simulink model "MicroMouseTemplate"  (R2024a)
settings: Solver=FixedStepAuto  StartTime=0.0  StopTime=10.0  RelTol=1e-3  EnableMultiTasking=on
undefined symbols (not defined in the file): samplingTime
settings Model: STM32="{\"DigitalPortWrite\":[{\"ID\":\"MicroMouseTemplate:84:3\"},{\"ID\":\"MicroMouseTemplate:84:4\"},{\"ID\":\"MicroMouseTemplate:84:5\"},{\"ID\":\"MicroMouseTemplate:84:6\"},{\"ID\":\"MicroMouseTemplate:84:7\"},{\"ID\":\"MicroMouseTemplate:84:8\"},{\"ID\":\"MicroMouseTemplate:84:9\"},{\"ID\":\"MicroMouseTemplate:84:10\"},{\"ID\":\"MicroMouseTemplate:160:19\"},{\"ID\":\"MicroMouseTemplate:2479:4\"},{\"ID\":\"MicroMouseTemplate:2479:6\"},{\"ID\":\"MicroMouseTemplate:2479:7\"},{\"ID\":\"MicroMouseTemplate:2479:8\"}],\"PWMOutput\":[{\"ID\":\"MicroMouseTemplate:160:24\"},{\"ID\":\"MicroMouseTemplate:160:25\"}],\"AnalogInput\":{\"ID\":\"MicroMouseTemplate:2357:1\"},\"DigitalPortRead\":[{\"ID\":\"MicroMouseTemplate:2483:3\"},{\"ID\":\"MicroMouseTemplate:2483:4\"}]}"  ExtModeTrigDuration=10  Creator=JesseJabezArendse  LastModifiedBy=griff
settings SolverCC: AllowMultiTaskInputOutput=on  AutoInsertRateTranBlk=on  InsertRTBMode=Never (minimum delay)
settings OptimizationCC: EnhancedBackFolding=on  PassReuseOutputArgsAs=Individual arguments  StateBitsets=on  DataBitsets=on  ZeroExternalMemoryAtStartup=off  ZeroInternalMemoryAtStartup=off  NoFixptDivByZeroProtection=on  MaxStackSize=64  OptimizeBlockOrder=speed  DifferentSizesBufferReuse=on  EfficientTunableParamExpr=on
settings DebuggingCC: MultiTaskCondExecSysMsg=none  ParameterOverflowMsg=none  ParameterPrecisionLossMsg=none  ParameterTunabilityLossMsg=error
settings HardwareCC: ProdBitPerPointer=32  ProdBitPerSizeT=32  ProdBitPerPtrDiffT=32  ProdLargestAtomicInteger=Long  ProdLargestAtomicFloat=Double  ProdWordSize=32  ProdLongLongMode=on  ProdHWDeviceType=ARM Compatible->ARM Cortex  TargetBitPerPointer=64  TargetBitPerSizeT=64  TargetBitPerPtrDiffT=64  TargetLongLongMode=on  TargetIntDivRoundTo=Zero  TargetEndianess=LittleEndian  TargetWordSize=64  TargetHWDeviceType=MATLAB Host
settings ModelReferenceCC: EnableParallelModelReferenceBuilds=on  ParallelModelReferenceMATLABWorkerInit=Copy Base Workspace  SupportModelReferenceSimTargetCustomCode=on
settings SFSimCC: MATLABDynamicMemAlloc=off  SimHardwareAcceleration=native
settings RTWCC: Description=Embedded Coder  SystemTargetFile=ert.tlc  HardwareBoard=STM32L4xx Based  TLCOptions=-p0 -aInlineSetEventsForThisBaseRateFcn=TLC_FALSE -aSuppressMultiTaskScheduler=TLC_FALSE -aRateBasedStepFcn=1  TemplateMakefile=ert_default_tmf  Toolchain=GNU Tools for ARM Embedded Processors  BuildConfiguration=Faster Runs  CodeExecutionProfiling=on  CodeProfilingInstrumentation=coarse  GPUComputeCapability=3.5
settings RTWCC: CustomHeaderCode=|
  | #include "MicroMouseProgramming\Core\Inc\IMU.h"
  | #include "MicroMouseProgramming\Core\Inc\CustomWhile.h"
  | #include "MicroMouseProgramming\Core\Inc\Motors.h"
settings RTWCC: CustomInclude=|
  | MicroMouseProgramming\Core\Inc\
  | MicroMouseProgramming\Core\Src\
settings RTWCC: CustomSource=|
  | MicroMouseProgramming\Core\Src\IMU.c
  | MicroMouseProgramming\Core\Src\CustomWhile.c
  | MicroMouseProgramming\Core\Src\Motors.c
settings CodeAppCC: GenerateComments=off  IgnoreCustomStorageClasses=off  OperatorAnnotations=on  SimulinkDataObjDesc=on  SFDataObjDesc=on  SimulinkBlockComments=off
settings ERTTargetCC: CodeReplacementLibrary=ARM Cortex-M  SupportNonFinite=off  SupportComplex=off  SupportVariableSizeSignals=on  ExtModeTransport=3  ExtModeStaticAlloc=on  ExtModeStaticAllocSize=2048  ExtModeMexFile=ext_xcp  ExtModeIntrfLevel=Level2 - Open

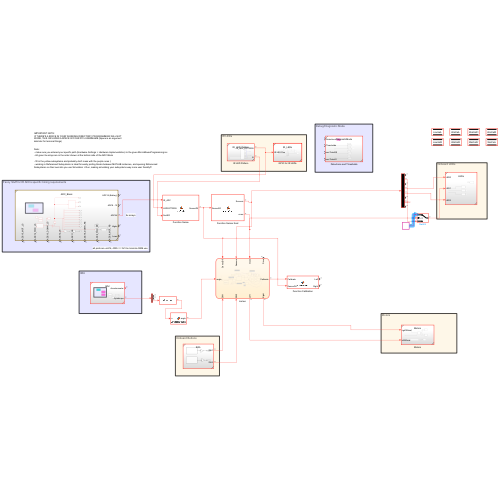
[thumbnail: Simulink's stored preview of the top-level diagram]
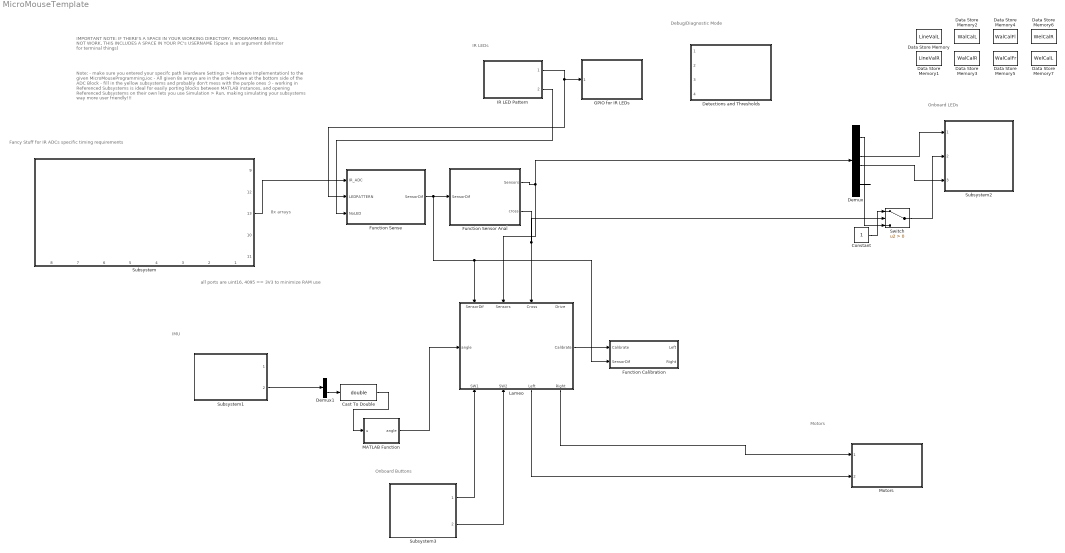
== system MicroMouseTemplate ==
  note: IMPORTANT NOTE:
      | IF THERE'S A SPACE IN YOUR WORKING DIRECTORY, PROGRAMMING WILL NOT WORK, THIS INCLUDES A SPACE IN YOUR PC's USERNAME (Space is an argument delimiter for terminal things)
  note: Note:
      | - make sure you entered your specifc path (Hardware Settings > Hardware Implementation) to the given MicroMouseProgramming.ioc
      | - All given 8x arrays are in the order shown at the bottom side of the ADC Block
      |
      | - fill in the yellow subsystems and probably don't mess with the purple ones :)
      | - working in Referenced Subsystems is ideal for easily porting blocks between MATLAB instances, and opening Referenced Subsystems on their own lets you use Simulation > Run, making simulating your subsystems way more user friendly!!!
  note: 8x arrays
  note: all ports are uint16, 4095 == 3V3 to minimize RAM use
  note: IMU
  note: Fancy Stuff for IR ADCs specific timing requirements
  note: IR LEDs
  note: Motors
  note: Onboard Buttons
  note: Onboard LEDs
  note: Debug/Diagnostic Mode
  Cast To Double : DataTypeConversion  OutDataTypeStr=double  SaturateOnIntegerOverflow=off  RndMeth=Floor
  Constant : Constant
  Data Store Memory : DataStoreMemory  DataStoreName=LineValL  WriteAfterWriteMsg=warning  ShowAdditionalParam=off  OutDataTypeStr=double
  Data Store Memory1 : DataStoreMemory  DataStoreName=LineValR  WriteAfterWriteMsg=warning  ShowAdditionalParam=off  OutDataTypeStr=double
  Data Store Memory2 : DataStoreMemory  DataStoreName=WalCalL  WriteAfterWriteMsg=warning  ShowAdditionalParam=off  OutDataTypeStr=double
  Data Store Memory3 : DataStoreMemory  DataStoreName=WalCalR  WriteAfterWriteMsg=warning  ShowAdditionalParam=off  OutDataTypeStr=double
  Data Store Memory4 : DataStoreMemory  DataStoreName=WalCalFl  WriteAfterWriteMsg=warning  ShowAdditionalParam=off  OutDataTypeStr=double
  Data Store Memory5 : DataStoreMemory  DataStoreName=WalCalFr  WriteAfterWriteMsg=warning  ShowAdditionalParam=off  OutDataTypeStr=double
  Data Store Memory6 : DataStoreMemory  DataStoreName=WelCalR  WriteAfterWriteMsg=warning  ShowAdditionalParam=off  OutDataTypeStr=double
  Data Store Memory7 : DataStoreMemory  DataStoreName=WelCalL  WriteAfterWriteMsg=warning  ShowAdditionalParam=off  OutDataTypeStr=double
  Demux : Demux  Outputs=8
  Demux1 : Demux  Outputs=3
  Detections and Thresholds : Subsystem  ReferencedSubsystem=DiagnosticMode
  Function Calibration : MATLAB Function  TreatAsAtomicUnit=on
  Function Sense : MATLAB Function  TreatAsAtomicUnit=on
  Function Sensor Anal : MATLAB Function  TreatAsAtomicUnit=on
  GPIO for IR LEDs : Subsystem  TreatAsAtomicUnit=on  SystemSampleTime=samplingTime  ReferencedSubsystem=IR_LEDs
  IR LED Pattern : Subsystem  ReferencedSubsystem=IR_LED_Pattern
  Lameo : Stateflow chart  TreatAsAtomicUnit=on
      settings: PortSchema="{\"entries\":[{\"content\":{\"sides\":[{\"content\":{\"connectorIds\":[\"In2\"]},\"type\":\"ConnectorPlacement.EquallySpacedRectSide\",\"uuid\":\"f52daa4f-6374-42e5-9ef1-0ccc99d09b58\"},{\"content\":{\"connectorIds\":[\"Out1\"],\"side\":\"RIGHT\"},\"type\":\"ConnectorPlacement.EquallySpacedRectSide\",\"uuid\":\"94b478cc-4dde-45c7-a588-77cf2b43cdb7\"},{\"content\":{\"connectorIds\":[\"In1\",\"In3\",\"In4\",\"Out2\"],\"side\":\"TOP\"},\"type\":\"ConnectorPlacement.EquallySpacedRectSide\",\"uuid\":\"afff2079-ea5c-423e-9722-09c3bbce433b\"},{\"content\":{\"connectorIds\":[\"In6\",\"In5\",\"Out3\",\"Out4\"],\"side\":\"BOTTOM\"},\"type\":\"ConnectorPlacement.EquallySpacedRectSide\",\"uuid\":\"94e93a1d-795d-41a3-b2d8-d520b2bf47ef\"}]},\"type\":\"ConnectorPlacement.EquallySpacedConnector\",\"uuid\":\"d4d35636-54af-48ac-af70-d56caef5e090\"}],\"packageUris\":[\"http://schema.mathworks.com/mf0/Connector/R2020b\"],\"version\":\"1.0\"}"
  MATLAB Function : MATLAB Function  TreatAsAtomicUnit=on
  Motors : Subsystem  ReferencedSubsystem=Motors
  Subsystem : Subsystem  ReferencedSubsystem=ADC_Block
      settings: PortSchema="{\"entries\":[{\"content\":{\"sides\":[{\"content\":{},\"type\":\"ConnectorPlacement.EquallySpacedRectSide\",\"uuid\":\"be6b81d5-7a49-4e34-b35f-0c07892094fc\"},{\"content\":{\"connectorIds\":[\"Out1\",\"Out2\",\"Out3\",\"Out4\",\"Out5\",\"Out6\",\"Out7\",\"Out8\"],\"side\":\"RIGHT\"},\"type\":\"ConnectorPlacement.EquallySpacedRectSide\",\"uuid\":\"5e22590a-b7c0-4c63-8de4-8d81fd6c3849\"},{\"content\":{\"connectorIds\":[\"Out9\",\"Out12\",\"Out13\",\"Out10\",\"Out11\"],\"side\":\"TOP\"},\"type\":\"ConnectorPlacement.EquallySpacedRectSide\",\"uuid\":\"da97636e-cea0-4a10-8fe5-d807f9ee999f\"},{\"content\":{\"side\":\"BOTTOM\"},\"type\":\"ConnectorPlacement.EquallySpacedRectSide\",\"uuid\":\"a593d780-81a8-4730-a8bc-2bbf356cafe4\"}]},\"type\":\"ConnectorPlacement.EquallySpacedConnector\",\"uuid\":\"0bcac921-e51a-4437-9183-315712d0a8c2\"}],\"packageUris\":[\"http://schema.mathworks.com/mf0/Connector/R2020b\"],\"version\":\"1.0\"}"
  Subsystem1 : Subsystem  ReferencedSubsystem=IMU
  Subsystem2 : Subsystem  ReferencedSubsystem=LEDs
  Subsystem3 : Subsystem  ReferencedSubsystem=SWs
  Switch : Switch  Criteria=u2 > Threshold  SaturateOnIntegerOverflow=off  InputSameDT=off
  wires:
  Subsystem3/1 -> Lameo/6(SW1)
  Subsystem3/2 -> Lameo/5(SW2)
  IR LED Pattern/1 -> Function Sense/2(LEDPATTERN), GPIO for IR LEDs/1
  Subsystem/13 -> Function Sense/1(IR_ADC)
  IR LED Pattern/2 -> Function Sense/3(NoLED)
  Function Sense/1(SensorDif) -> Lameo/1(SensorDif), Function Calibration/2(SensorDif), Function Sensor Anal/1(SensorDif)
  Lameo/1(Calibrate) -> Function Calibration/1(Calibrate)
  Lameo/3(Left) -> Motors/2
  Lameo/4(Right) -> Motors/1
  Function Sensor Anal/1(Sensors) -> Lameo/3(Sensors), Demux/1
  Function Sensor Anal/2(cross) -> Switch/2, Lameo/4(Cross)
  Subsystem1/2 -> Demux1/1
  Demux1/3 -> Cast To Double/1
  Cast To Double/1 -> MATLAB Function/1(u)
  MATLAB Function/1(angle) -> Lameo/2(angle)
  Demux/2 -> Switch/3
  Demux/7 -> ?
  Demux/4 -> Subsystem2/1
  Demux/5 -> Subsystem2/3
  Constant/1 -> Switch/1
  Switch/1 -> Subsystem2/2

== matlab function MicroMouseTemplate/Function Calibration ==
  data: Calibrate input; Left output; Right output; LineValR data_store_memory; SensorDif input; LineValL data_store_memory; WalCalR data_store_memory; WalCalL data_store_memory; WalCalFr data_store_memory; WalCalFl data_store_memory; WelCalL data_store_memory; WelCalR data_store_memory
function [Left,Right]  = Calbiration(Calibrate, SensorDif)


persistent mindl
if isempty(mindl)
    mindl = 3;
end
persistent maxdl
if isempty(maxdl)
    maxdl = 0;
end
persistent mindr
if isempty(mindr)
    mindr = 3;
end
persistent maxdr
if isempty(maxdr)
    maxdr = 0;
end



persistent minwl
if isempty(minwl)
    minwl = 3;
end
persistent maxwl
if isempty(maxwl)
    maxwl = 0;
end

persistent minwfr
if isempty(minwfr)
    minwfr = 3;
end
persistent maxwfr
if isempty(maxwfr)
    maxwfr = 0;
end
persistent minwfl
if isempty(minwfl)
    minwfl = 3;
end
persistent maxwfl
if isempty(maxwfl)
    maxwfl = 0;
end

persistent minwr
if isempty(minwr)
    minwr = 3;
end
persistent maxwr
if isempty(maxwr)
    maxwr = 0;
end

persistent minwer
if isempty(minwer)
    minwer = 3;
end
persistent maxwer
if isempty(maxwer)
    maxwer = 0;
end
persistent minwel
if isempty(minwel)
    minwel = 3;
end
persistent maxwel
if isempty(maxwel)
    maxwel = 0;
end






Left=0;
Right=0;
if Calibrate==1
    Right=75;
    Left=-75;
    if SensorDif(3)>(maxdl)
        maxdl=maxdl*0.8+0.2*SensorDif(3);
    end
    if SensorDif(3)<(mindl)
        mindl=mindl*0.8+0.2*SensorDif(3);
    end
    if SensorDif(6)>(maxdr)
        maxdr=maxdr*0.8+0.2*SensorDif(6);
    end
    if SensorDif(6)<(mindr)
        mindr=mindr*0.8+0.2*SensorDif(6);
    end

    if SensorDif(4)>(maxwr)
        maxwr=maxwr*0.5+0.5*SensorDif(4);
    end
    if SensorDif(4)<(minwr)
        minwr=minwr*0.5+0.5*SensorDif(4);
    end
    if SensorDif(5)>(maxwl)
        maxwl=maxwl*0.5+0.5*SensorDif(5);
    end
    if SensorDif(5)<(minwl)
        minwl=minwl*0.5+0.5*SensorDif(5);
    end

    if (SensorDif(2))>(maxwfr)
        maxwfr=maxwfr*0.5+0.5*(SensorDif(2));
    end
    if (SensorDif(2))<(minwfr)
        minwfr=minwfr*0.5+0.5*(SensorDif(2));
    end
    if (SensorDif(7))>(maxwfl)
        maxwfl=maxwfl*0.5+0.5*(SensorDif(7));
    end
    if (SensorDif(7))<(minwfl)
        minwfl=minwfl*0.5+0.5*(SensorDif(7));
    end


     if SensorDif(1)>(maxwer)
        maxwer=maxwer*0.8+0.2*SensorDif(1);
    end
    if SensorDif(1)<(minwer)
        minwer=minwer*0.8+0.2*SensorDif(1);
    end
    if SensorDif(8)>(maxwel)
        maxwel=maxwel*0.8+0.2*SensorDif(8);
    end
    if SensorDif(8)<(minwel)
        minwel=minwel*0.8+0.2*SensorDif(8);
    end


end



global LineValR
LineValR=(maxdr-mindr)*0.7+mindr;%(mindr+maxdr)/2*1.1;
global LineValL
LineValL=(maxdl-mindl)*0.7+mindl;%(mindl+maxdl)/2*1.1;

global WalCalL
WalCalL=(maxwl-minwl)*0.4+minwl;%(minwl+maxwl)/2;
%WalCalL=((maxwl)*0.85);
global WalCalR
WalCalR=(maxwr-minwr)*0.4+minwr;%(minwr+maxwr)/2;
%WalCalR=((maxwr)*0.85);
global WalCalFl
%WalCalFl=(minwfl+maxwfl)/2;
WalCalFl=(maxwfl-minwfl)*0.3+minwfl;%((maxwfl)*0.6);
global WalCalFr
%WalCalFr=(minwfr+maxwfr)/2;
WalCalFr=(maxwfr-minwfr)*0.3+minwfr;%((maxwfr)*0.6);

global WelCalL
WelCalL=(maxwel-minwel)*0.8+minwel;
global WelCalR
WelCalR=(maxwer-minwer)*0.8+minwer;

end

== stateflow chart MicroMouseTemplate/Lameo ==
  state Crossing
    entry:
    Turn =thingy;
    pos(1)=pos(1)+direction(2)-direction(4);
    pos(2)=pos(2)+direction(1)-direction(3);
  state Calibration
    during:
    Calibrate =1 ;
    Right=50;
    Left=-50;
  state Delay
  state Center
    during:
    [Left,Right]=CenterLine(1,Sensors)
    Calibrate =0;
  state Back
    during:
    Left=-50;
    Right=-50;
  state Back2
    during:
    Left=-50;
    Right=-50;
  state Back1
    during:
    Left=-50;
    Right=-50;
  state OK
    entry:
    temp=start
    start=dest
    dest=temp
    Left=0;
    Right=0;
  state TurnRight
    entry:
    Left=100;
    Right=-50;
    DesA=angle-90;
    exit:
    Left=0;
    Right=0;
    res=1;
  state TurnLeft
    entry:
    Left=-50;
    Right=100;
    DesA=angle+90;
    exit:
    Left=0;
    Right=0;
    res=1;
  state Flip
    entry:
    Left=-50;
    Right=50;
    DesA=angle+180;
    exit:
    Left=0;
    Right=0;
    res=1;
  state Idle
    entry:
    %Varibales needed for path finding
    Left=0;
    Right=0;
    pathend=0;
    %end
    during:
    Calibrate =0 ;
    Drive=0;
  state Drive
    entry:
    Drive=1;
    [Left,Right]=FollowLine(Drive,Sensors,res,SensorDif)
    during:
    [Left,Right]=FollowLine(Drive,Sensors,0,SensorDif)
  state Init1
    entry:
    Init;
    start=int16([1;1]);
    pos=start;
    dest=int16([2;1]);
    direction= int16([1;0;0;0]);
    desA=0;
  state Wait
  state TurnWrong
    entry:
    Left=-50;
    Right=50;
    exit:
    Left=0;
    Right=0;
  state TurnWrong1
    entry:
    Left=50;
    Right=-50;
    exit:
    Left=0;
    Right=0;
  state TurnWrong2
    entry:
    Left=50;
    Right=-50;
    exit:
    Left=0;
    Right=0;
  state Hehehehe
    state T
      during:
      Left=100;
      Right=-100;
    state TT
      during:
      Left=-100;
      Right=100;
    (default) -> T
    TT -> T : after(0.02,sec)
    T -> TT : after(0.02,sec)
  state Mistake
    entry:
    delConnection(pos(1),pos(2),pos(1)+direction(2)-direction(4),pos(2)+direction(1)-direction(3))
    direction= circshift(direction,2);
    pos(1)=pos(1)+direction(2)-direction(4);
    pos(2)=pos(2)+direction(1)-direction(3)
  state TEst
    entry:
    desA=desA+90;
    during:
    [Left,Right]=CenterAngle(angle,desA)
  OK -> Delay : after(2,sec)
  Delay -> Crossing : after(1,sec)
  Crossing -> Back [order 3] : [Turn==2]
  Calibration -> Center : [after(4,sec)]
  Crossing -> Back1 [order 1] : [Turn==-1]
  Idle -> Delay [order 2] : [SW1]
  Crossing -> Back2 [order 2] : [Turn==1]
  Idle -> Calibration [order 1] : [SW2&&after(2,sec)]
  Drive -> Crossing [order 2] : [Cross==1&&(after(0.4,sec))]
  (default) -> Wait
  Back -> Flip : after(0.1,sec)
  Back2 -> TurnRight : after(0.1,sec)
  Back1 -> TurnLeft : after(0.1,sec)
  Center -> Idle : after(1,sec)
  Crossing -> Drive [order 4] : [Turn==0]{res=0;}
  Drive -> OK [order 1] : [Cross==1&&(after(0.4,sec))&&(pos(1)==dest(1)&&pos(2)==dest(2))]
  Mistake -> Flip
  TurnRight -> TurnWrong : [(DesA-angle>-20)&&Sensors(6)==0]
  TurnLeft -> TurnWrong1 : [(DesA-angle<20)&&Sensors(3)==0]
  Flip -> TurnWrong2 : [(DesA-angle<10)&&Sensors(6)==0]
  Wait -> Init1 : after(1,sec)
  TurnWrong -> Drive : after(0.05,sec)
  TurnWrong1 -> Drive : after(0.05,sec)
  Hehehehe -> Init1 : after(1,sec)
  TurnWrong2 -> Drive : after(0.1,sec)
  Init1 -> Idle
  Drive -> Mistake [commented out] : [Sensors(2)==1&&before(0.3,sec)]
  TEst -> TEst : after(1,sec)
  data: Drive function_input; Sensors function_input; Left function_output; Right function_output; Drive function_input; Sensors function_input; Left function_output; Right function_output; first function_input; SensorDif function_input; x1 function_input; y1 function_input; x2 function_input; y2 function_input; Angle function_input; Setpoint function_input; Left function_output; Right function_output; Turn function_output; SensorDif input; angle input; Sensors input; Cross input; SW2 input; SW1 input; Calibrate output; Drive output; Left output; Right output; Turn local; numH local int16 size=1; numV local int16 size=1; pos local int16 size=2; dest local int16 size=2; direction local int16 size=4; connection local int16 size=168 4; connectionend local int16 size=1; dist local int16 size=[7 7]; path local int16 size=200 2; pre local int16 size=7 7 2; q local int16 size=200 2; qend local int16 size=1; pathend local int16 size=1; start local; temp local; desA local; DesA local; LineValR data_store_memory; LineValL data_store_memory; res local
  function [Left,Right] = CenterLine(Drive, Sensors):
    | function [Left,Right] = CenterLine(Drive, Sensors)
    | P = 10;
    | I =0.5;
    | D=50;
    | 
    | 
    | persistent preError
    | if isempty(preError)
    |     preError=0;
    | end
    | persistent sumError
    | if isempty(sumError)
    |     sumError=0;
    | end
    | persistent error
    | if isempty(error)
    |     error=0;
    | end
    | persistent Dave
    | if isempty(Dave)
    |     Dave=0;
    | end
    | 
    | 
    | 
    | Left=0;
    | Right=0;
    | 
    | if Drive ==1
    | Left=0;
    | Right=0;
    | 
    | 
    | if (Sensors(3)==1&&Sensors(6)==0)
    |     error=-1;   
    | end
    | if (Sensors(3)==0&&Sensors(6)==1)
    |     error=1;   
    | end
    | if (Sensors(3)==0&&Sensors(6)==0)
    |     error=0;   
    | end
    | if (error==1&&Sensors(3)==1&&Sensors(6)==1)
    |     error=2;  
    | end
    | if (error==-1&&Sensors(3)==1&&Sensors(6)==1)
    |     error=-2; 
    | end
    | 
    | sumError=sumError+error;
    | sumError= sumError-0.005*sumError;
    | 
    | 
    | Dave=(error-preError)+0.8*Dave;
    | 
    | PID= P*error+I*sumError+D*(Dave);
    | preError=error;
    | 
    | 
    | Left=0-PID;
    | Right=0+PID;
    | Left = min(max(Left,-100),100);
    | Right = min(max(Right,-100),100);
    | 
    | if (error==0&&Sensors(3)==1&&Sensors(6)==1)
    |     Left=-50;
    |     Right=-50;
    | end
    | 
    | 
    | 
    | 
    | 
    | if Sensors(2)==1
    |    % Left=0;
    |    % Right=0;
    | end
    | 
    | 
    | 
    | 
    | 
    | 
    | 
    | 
    | 
    | 
    | 
    | 
    | 
    | 
    | end
    | 
    | end
  function [Left,Right] = FollowLine(Drive, Sensors,first,SensorDif):
    | function [Left,Right] = FollowLine(Drive, Sensors,first,SensorDif)
    | P = 15;
    | I =0.5;
    | D=125;
    | global LineValL
    | global LineValR
    | 
    | 
    | 
    | persistent preError
    | if isempty(preError)
    |     preError=0;
    | end
    | persistent preSide
    | if isempty(preSide)
    |     preSide=0;
    | end
    | persistent sumError
    | if isempty(sumError)
    |     sumError=0;
    | end
    | persistent error
    | if isempty(error)
    |     error=0;
    | end
    | persistent Dave
    | if isempty(Dave)
    |     Dave=0;
    | end
    | 
    | if (first==1)
    |     Dave=0;
    |     error=0;
    |     preError=0;
    |     sumError=0;
    | end
    | 
    | Left=0;
    | Right=0;
    | 
    | if Drive ==1
    | Left=100;
    | Right=100;
    | 
    | 
    | if (Sensors(3)==1&&Sensors(6)==0)
    |     error=-1;  
    |     preSide = error;
    | end
    | if (Sensors(3)==0&&Sensors(6)==1)
    |     error=1;  
    |     preSide = error;
    | end
    | if (Sensors(3)==0&&Sensors(6)==0)
    |     error=0; 
    |    
    | end
    | if (error==1&&Sensors(3)==1&&Sensors(6)==1)
    |     error=2;  
    |     preSide = error;
    | end
    | if (error==-1&&Sensors(3)==1&&Sensors(6)==1)
    |     error=-2; 
    |     preSide = error;
    | end
    | 
    | if (error==0&&Sensors(3)==1&&Sensors(6)==1)
    |     error=-preSide;
    | end
    | 
    | 
    | sumError=sumError+error;
    | sumError= sumError-0.005*sumError;
    | 
    | 
    | Dave=(error-preError)+0.8*Dave;
    | 
    | PID= P*error+I*sumError+D*(Dave);
    | preError=error;
    | 
    | 
    | Left=100-PID;
    | Right=100+PID;
    | Left = min(max(Left,-100),100);
    | Right = min(max(Right,-100),100);
    | 
    | 
    | 
    | 
    | 
    | 
    | if Sensors(2)==1
    |    % Left=0;
    |    % Right=0;
    | end
    | 
    | 
    | 
    | 
    | 
    | 
    | 
    | 
    | 
    | 
    | 
    | 
    | 
    | 
    | end
    | 
    | end
  function Init:
    | function Init
    | global pos
    |  pos=int16([1;2]);
    |  global dest
    | dest=int16([2;1]);
    | global direction
    | direction= int16([1;0;0;0]);
    | global numH
    | numH = int16(7);
    | global numV
    | numV = int16(7);
    | global connection
    | connection = zeros(168,4,'int16');
    | global connectionend
    | connectionend=int16(0);
    | 
    | 
    | 
    | 
    | 
    | for x = 1:numH
    |        for y = 1:numV
    |             if x>1
    |             connection(connectionend+1, :) = [x, y, x-1, y];
    |             connectionend=connectionend+1;
    |             end
    |             if y>1
    |              connection(connectionend+1, :) = [x, y, x, y-1];
    |              connectionend=connectionend+1;
    |             end
    |             if x<numH
    |              connection(connectionend+1, :) = [x, y, x+1, y];
    |              connectionend=connectionend+1;
    |             end
    |             if y<numV
    |              connection(connectionend+1, :) = [x, y, x, y+1];
    |              connectionend=connectionend+1;
    |             end
    | 
    | 
    |        end
    | end
    | 
    | end
  function delConnection(x1,y1,x2,y2):
    | function delConnection(x1,y1,x2,y2)
    | global connection;
    |     for i = 1:size(connection,1)
    |         if connection(i,1) == x1 & connection(i,2) == y1 & connection(i,3) == x2 & connection(i,4) == y2
    |             connection(i,:) = [0,0,0,0];
    |         end
    |         if connection(i,1) == x2 & connection(i,2) == y2 & connection(i,3) == x1 & connection(i,4) == y1
    |             connection(i,:) = [0,0,0,0];
    |         end
    |         
    |     end
    | 
    | end
  function route:
    | function route
    |     global connection;
    |     global dist;
    |     global pre;
    |     global q;
    |     global qend;
    | 
    |     global pos;
    |     global path;
    |     global pathend;
    |     global dest;
    | 
    | dist = (zeros(7,7,'int16')+inf);
    | pre = zeros(7,7,2,'int16');
    | q= zeros(200,2,'int16');
    | qend=int16(0);
    | path= zeros(200,2,'int16');
    | pathend=int16(0);
    | dist(pos(1),pos(2))=0;
    | q(qend+1,:)=[pos(1), pos(2)];
    | qend=qend+1;
    | 
    | 
    | while qend>0
    |     x1 = q(1,1);
    |     y1 =q(1,2);
    | 
    |         for i = 1:size(connection,1)
    |             if connection(i,1) == x1 & connection(i,2) == y1 
    |                 if dist(connection(i,3), connection(i,4))> (dist(x1,y1)+1)
    |                     dist(connection(i,3), connection(i,4))= dist(x1,y1)+1;
    |                     pre(connection(i,3), connection(i,4),:)=[x1,y1];
    |                     q(qend+1,:)=[connection(i,3),connection(i,4)];
    |                     qend=qend+1;
    |                 end
    |     
    |             end
    |             
    |             
    |         end
    |         for i=1:1:(qend-1)
    |             q(i,:)=q(i+1,:);
    |         end
    |          qend=qend-1;
    | end
    | 
    | %convert pre map to path
    | q=zeros(200,2,'int16');
    | qend=int16(0);
    | q(qend+1,:)=[dest(1), dest(2)];
    | qend=qend+1;
    | hold on;
    | 
    | %path= zeros(200,2,'int16');
    | while q(1,1)>0
    |     path(pathend+1,:) = q(1,:);
    |     pathend=pathend+1;
    |     q(qend+1,:)=pre(q(1,1), q(1,2),:);
    |     qend=qend+1;
    |         for i=1:1:(size(q,1)-1)
    |             q(i,:)=q(i+1,:);  
    |         end
    |         qend=qend-1;
    | end
    |             
    | 
    | end
  function [Left,Right] = CenterAngle(Angle,Setpoint):
    | function [Left,Right] = CenterAngle(Angle,Setpoint)
    | P = 2;
    | I =0.02;
    | D=8;
    | 
    | 
    | persistent preError
    | if isempty(preError)
    |     preError=0;
    | end
    | persistent sumError
    | if isempty(sumError)
    |     sumError=0;
    | end
    | persistent error
    | if isempty(error)
    |     error=0;
    | end
    | persistent Dave
    | if isempty(Dave)
    |     Dave=0;
    | end
    | 
    | 
    | 
    | 
    | 
    | 
    | error=Setpoint-Angle;
    | 
    | sumError=sumError+error;
    | sumError= sumError-0.005*sumError;
    | 
    | 
    | Dave=(error-preError)+0.8*Dave;
    | 
    | PID= P*error+I*sumError+D*(Dave);
    | preError=error;
    | 
    | 
    | Left=0-PID;
    | Right=0+PID;
    | Left = min(max(Left,-75),75);
    | Right = min(max(Right,-75),75);
    | 
    | 
    | 
    | 
    | 
    | 
    | 
    | 
    | 
    | 
    | 
    | 
    | 
    | 
    | 
    | 
    | 
    | 
    | 
    | 
    | 
    | 
    | end
  function Turn = thingy:
    | function Turn = thingy()
    | global Sensors
    | global path
    | global pathend
    | global pos
    | global direction
    | if Sensors(7)==1 || Sensors(2)
    |     delConnection(pos(1),pos(2),pos(1)+direction(2)-direction(4),pos(2)+direction(1)-direction(3))
    | end
    | if Sensors(5)==1 %right
    |     delConnection(pos(1),pos(2),pos(1)+direction(1)-direction(3),pos(2)+direction(4)-direction(2))
    | end
    | if Sensors(4)==1 %left
    |     delConnection(pos(1),pos(2),pos(1)+direction(3)-direction(1),pos(2)+direction(2)-direction(4))
    | end
    | 
    | 
    | %find best route on current knowledge
    |     route;
    |     Turn=0;
    |     if path(pathend-1,1)>pos(1) & direction(1) ==1
    |         Turn =1;
    |         direction= circshift(direction,1);
    |     end
    |     if path(pathend-1,1)>pos(1) & direction(3) ==1
    |         Turn=-1;
    |         direction= circshift(direction,-1);
    |     end
    |     if path(pathend-1,1)<pos(1) & direction(1) ==1
    |         Turn=-1;
    |         direction= circshift(direction,-1);
    |     end
    |     if path(pathend-1,1)<pos(1) & direction(3) ==1
    |         Turn=1;
    |         direction= circshift(direction,1);
    |     end
    | 
    |     %%%%%%%%
    |     if path(pathend-1,2)>pos(2) & direction(2) ==1
    |         Turn=-1;
    |         direction= circshift(direction,-1);
    |     end
    |     if path(pathend-1,2)>pos(2) & direction(4) ==1
    |         Turn=1;
    |         direction= circshift(direction,1);
    |     end
    |     if path(pathend-1,2)<pos(2) & direction(2) ==1
    |         Turn=1;
    |         direction= circshift(direction,1);
    |     end
    |     if path(pathend-1,2)<pos(2) & direction(4) ==1
    |         Turn=-1;
    |         direction= circshift(direction,-1);
    |     end
    | %%%%%%%
    |     if path(pathend-1,2)<pos(2) & direction(1) ==1
    |         Turn=2;
    |         direction= circshift(direction,2);
    |     end
    |     if path(pathend-1,2)>pos(2) & direction(3) ==1
    |        Turn=2;
    |        direction= circshift(direction,2);
    |     end
    |     if path(pathend-1,1)<pos(1) & direction(2) ==1
    |         Turn=2;
    |         direction= circshift(direction,2);
    |     end
    |     if path(pathend-1,1)>pos(1) & direction(4) ==1
    |         Turn=2;
    |         direction= circshift(direction,2);
    |     end
    | 
    |   
    |     
    |  
    | 
    | end

== matlab function MicroMouseTemplate/Function Sense ==
  data: IR_ADC input; LEDPATTERN input; SensorDif output; NoLED input
function SensorDif= SENSE(IR_ADC, LEDPATTERN, NoLED)
persistent prePAT;
if isempty(prePAT)
    prePAT = LEDPATTERN;
end
persistent preNoLED;
if isempty(preNoLED)
    preNoLED = NoLED;
end
persistent preDif;
if isempty(preDif)
    preDif = [0,0,0,0,0,0,0,0];
end



persistent ADCOFF;
if isempty(ADCOFF)
    ADCOFF = [0,0,0,0,0,0,0,0];
end
persistent ADCON;
if isempty(ADCON)
    ADCON = [0,0,0,0,0,0,0,0];
end

if preNoLED==1
    ADCOFF=IR_ADC;
end

for i = 1:8
    if prePAT(i)==1
        ADCON(i)=IR_ADC(i);
    end
    

end
SensorDif=preDif;
for i=1:8
    if prePAT(i)==1
    SensorDif(i)=  ADCON(i)-ADCOFF(i);
    end
end

   if prePAT(2)==1
        SensorDif(2)=(SensorDif(2)*2-preDif(2))*0.8+0.2*SensorDif(2);
   end
   if prePAT(4)==1
        SensorDif(4)=SensorDif(4)*1+0*preDif(4);
   end
   if prePAT(5)==1
        SensorDif(5)=SensorDif(5)*1+0*preDif(5);
   end
   if prePAT(7)==1
        SensorDif(7)=(SensorDif(7)*2-preDif(7))*0.8+0.2*SensorDif(7);
   end

preDif=SensorDif;



preNoLED=NoLED;
prePAT=LEDPATTERN;
end

== matlab function MicroMouseTemplate/Function Sensor Anal ==
  data: SensorDif input; Sensors output; LineValR data_store_memory; LineValL data_store_memory; WalCalFr data_store_memory; WalCalFl data_store_memory; WalCalR data_store_memory; WalCalL data_store_memory; WelCalL data_store_memory; WelCalR data_store_memory; cross output
function [Sensors,cross]  = SensorAnal(SensorDif)
Sensors=[0,0,0,0,0,0,0,0];
global LineValL
global LineValR
global WalCalFr
global WalCalFl
global WalCalR
global WalCalL
global WelCalR
global WelCalL

persistent sens8
if isempty(sens8)
    sens8=0;
end



if SensorDif(3)>LineValL
    Sensors(3)=1;
end
if SensorDif(6)>LineValR
    Sensors(6)=1;
end


if (SensorDif(2))>WalCalFr
    Sensors(2)=1;
end
if (SensorDif(7))>WalCalFl
    Sensors(7)=1;
end
if (SensorDif(5))>WalCalL
    Sensors(5)=1;
end
if (SensorDif(4))>WalCalR
    Sensors(4)=1;
end

if SensorDif(8)>WelCalL
    Sensors(8)=1;

end
if SensorDif(1)>WelCalR
   Sensors(1) =1;
end

if Sensors(8)<1 &&(SensorDif(6)+SensorDif(3))<(LineValR+LineValL)
    cross=1;
else
    cross=0;
end
sens8 = Sensors(8);

end

== matlab function MicroMouseTemplate/MATLAB Function ==
  data: u input; angle output
function angle = DirectionAngle(u)
persistent sum
if isempty(sum)
 sum =0;
end
sum =sum+u*0.01;
angle=sum;
end
